simulink model "Simulink_multiterminal_HVDC_grid_alphas"  (R2016a)
settings: Solver=ode4  StartTime=0.0  StopTime=tsimul  FixedStep=1e-5  MaxStep=1e-4  RelTol=1e-5
values from neighbouring files (symbols this model uses):
  c = 0.1616*(10^-6)    (= 1.616e-07)    [Parameters_multiterminal_HVDC_alphas.m]
  Cconv = 1.5*(10^-4)    (= 0.00015)    [Parameters_multiterminal_HVDC_alphas.m]
  d1 = 230    [Parameters_multiterminal_HVDC_alphas.m]
  d2 = 75    [Parameters_multiterminal_HVDC_alphas.m]
  d3 = 217    [Parameters_multiterminal_HVDC_alphas.m]
  E2ref = 640000    [Parameters_multiterminal_HVDC_alphas.m]
  Kp = 0.0017    [Parameters_multiterminal_HVDC_alphas.m]
  Kpdc1 = Kpdc*alpha    (= 0)    [Parameters_multiterminal_HVDC_alphas.m]
  Kpdc2 = Kpdc*(1-alpha)    (= 4000)    [Parameters_multiterminal_HVDC_alphas.m]
  l1 = 0.2644*(10^-3)    (= 0.0002644)    [Parameters_multiterminal_HVDC_alphas.m]
  l2 = 7.2865*(10^-3)    (= 0.0072865)    [Parameters_multiterminal_HVDC_alphas.m]
  l3 = 3.6198*(10^-3)    (= 0.0036198)    [Parameters_multiterminal_HVDC_alphas.m]
  Ll = 0.1956    [Parameters_multiterminal_HVDC_alphas.m]
  Qref = 0    [Parameters_multiterminal_HVDC_alphas.m]
  r1 = 0.1265    [Parameters_multiterminal_HVDC_alphas.m]
  r2 = 0.1504    [Parameters_multiterminal_HVDC_alphas.m]
  r3 = 0.0178    [Parameters_multiterminal_HVDC_alphas.m]
  Rg = (1/g)    (= 9852216.74877)    [Parameters_multiterminal_HVDC_alphas.m]
  rl = 3.072    [Parameters_multiterminal_HVDC_alphas.m]
  tau = 0.001    [Parameters_multiterminal_HVDC_alphas.m]
  taupll = 0.0045    [Parameters_multiterminal_HVDC_alphas.m]
  Uab = 320000    [Parameters_multiterminal_HVDC_alphas.m]
libraries: powerlib x115, simulink x4
(part 2 of 2)

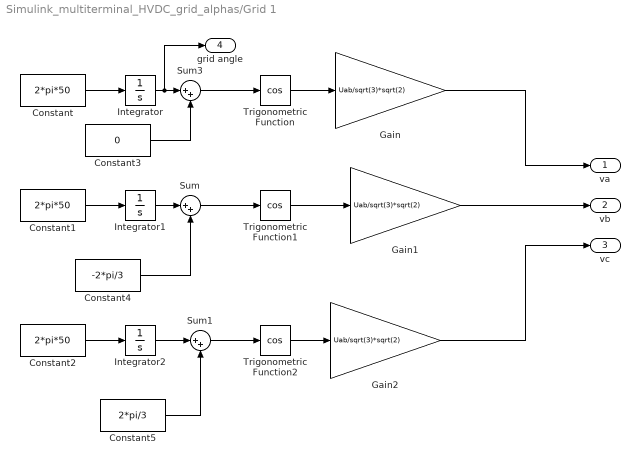
== system Simulink_multiterminal_HVDC_grid_alphas/Grid 1 ==
  Constant : Constant  Value=2*pi*50
  Constant1 : Constant  Value=2*pi*50
  Constant2 : Constant  Value=2*pi*50
  Constant3 : Constant  Value=0
  Constant4 : Constant  Value=-2*pi/3
  Constant5 : Constant  Value=2*pi/3
  Gain : Gain  Gain=Uab/sqrt(3)*sqrt(2)
  Gain1 : Gain  Gain=Uab/sqrt(3)*sqrt(2)
  Gain2 : Gain  Gain=Uab/sqrt(3)*sqrt(2)
  Integrator : Integrator
  Integrator1 : Integrator
  Integrator2 : Integrator
  Sum : Sum  Inputs=|++
  Sum1 : Sum  Inputs=|++
  Sum3 : Sum  Inputs=|++
  Trigonometric Function : Trigonometry  Operator=cos
  Trigonometric Function1 : Trigonometry  Operator=cos
  Trigonometric Function2 : Trigonometry  Operator=cos
  va : Outport
  vb : Outport  Port=2
  vc : Outport  Port=3
  grid angle : Outport  Port=4
  wires:
  Constant2/1 -> Integrator2/1
  Integrator2/1 -> Sum1/1
  Gain2/1 -> vc/1
  Sum1/1 -> Trigonometric Function2/1
  Sum3/1 -> Trigonometric Function/1
  Integrator/1 -> grid angle/1, Sum3/1
  Constant5/1 -> Sum1/2
  Constant4/1 -> Sum/2
  Integrator1/1 -> Sum/1
  Trigonometric Function/1 -> Gain/1
  Gain/1 -> va/1
  Constant1/1 -> Integrator1/1
  Trigonometric Function2/1 -> Gain2/1
  Constant/1 -> Integrator/1
  Constant3/1 -> Sum3/2
  Trigonometric Function1/1 -> Gain1/1
  Gain1/1 -> vb/1
  Sum/1 -> Trigonometric Function1/1

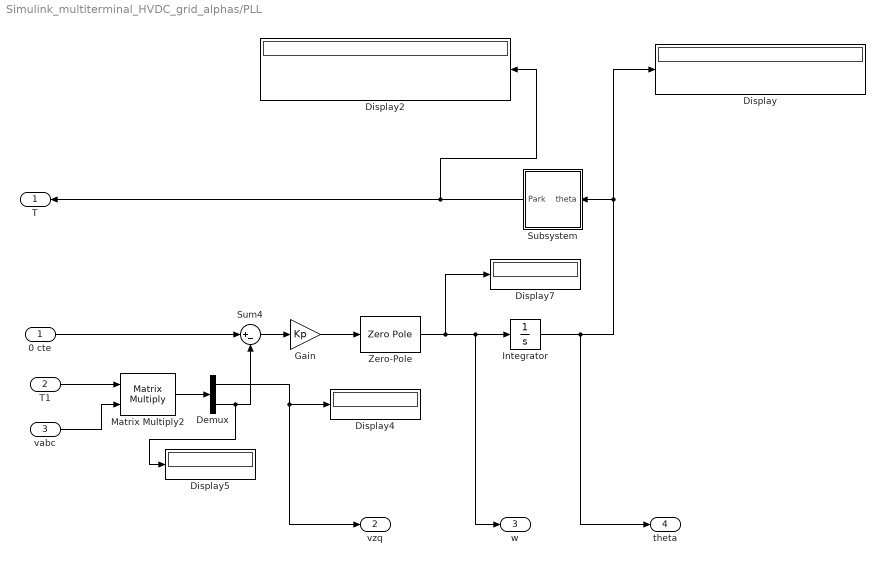
== system Simulink_multiterminal_HVDC_grid_alphas/PLL  ==
  0 cte : Inport
  T1 : Inport  Port=2
  vabc : Inport  Port=3
  Demux : Demux  Outputs=2
  Display{,2,4..5,7} (5 alike) : Display
  Gain : Gain  Gain=Kp
  Integrator : Integrator
  Matrix Multiply2 : Product  Multiplication=Matrix(*)
  Subsystem : Subsystem
  Sum4 : Sum  Inputs=|+-
  Zero-Pole : ZeroPole  Zeros=[-1/taupll]  Poles=[0]
  T : Outport
  vzq : Outport  Port=2
  w : Outport  Port=3
  theta : Outport  Port=4
  wires:
  0 cte/1 -> Sum4/1
  Subsystem/1(Park) -> T/1, Display2/1
  Sum4/1 -> Gain/1
  Gain/1 -> Zero-Pole/1
  Zero-Pole/1 -> Display7/1, w/1, Integrator/1
  Integrator/1 -> theta/1, Display/1, Subsystem/1(theta)
  T1/1 -> Matrix Multiply2/1
  vabc/1 -> Matrix Multiply2/2
  Matrix Multiply2/1 -> Demux/1
  Demux/2 -> Display5/1, Sum4/2
  Demux/1 -> vzq/1, Display4/1

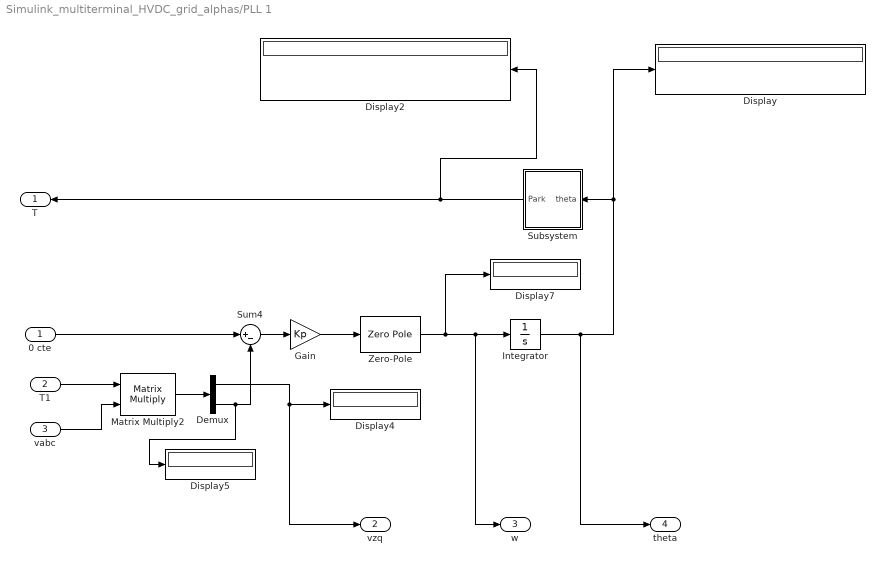
== system Simulink_multiterminal_HVDC_grid_alphas/PLL 1 ==
  0 cte : Inport
  T1 : Inport  Port=2
  vabc : Inport  Port=3
  Demux : Demux  Outputs=2
  Display{,2,4..5,7} (5 alike) : Display
  Gain : Gain  Gain=Kp
  Integrator : Integrator
  Matrix Multiply2 : Product  Multiplication=Matrix(*)
  Subsystem : Subsystem
  Sum4 : Sum  Inputs=|+-
  Zero-Pole : ZeroPole  Zeros=[-1/taupll]  Poles=[0]
  T : Outport
  vzq : Outport  Port=2
  w : Outport  Port=3
  theta : Outport  Port=4
  wires:
  0 cte/1 -> Sum4/1
  Subsystem/1(Park) -> T/1, Display2/1
  Sum4/1 -> Gain/1
  Gain/1 -> Zero-Pole/1
  Zero-Pole/1 -> Display7/1, w/1, Integrator/1
  Integrator/1 -> theta/1, Display/1, Subsystem/1(theta)
  T1/1 -> Matrix Multiply2/1
  vabc/1 -> Matrix Multiply2/2
  Matrix Multiply2/1 -> Demux/1
  Demux/2 -> Display5/1, Sum4/2
  Demux/1 -> vzq/1, Display4/1

== system Simulink_multiterminal_HVDC_grid_alphas/Pac ==
  iabc : Inport
  vabc : Inport  Port=2
  Add : Sum  Inputs=+++
  Demux3 : Demux  Outputs=3
  Demux4 : Demux  Outputs=3
  Display23 : Display
  Product7 : Product
  Product8 : Product
  Product9 : Product
  Pac : Outport
  wires:
  vabc/1 -> Demux4/1
  Product7/1 -> Add/1
  Demux3/1 -> Product7/1
  Demux3/3 -> Product8/1
  Product9/1 -> Add/2
  Add/1 -> Pac/1, Display23/1
  Demux4/3 -> Product8/2
  Demux3/2 -> Product9/1
  Product8/1 -> Add/3
  Demux4/1 -> Product7/2
  Demux4/2 -> Product9/2
  iabc/1 -> Demux3/1

== system Simulink_multiterminal_HVDC_grid_alphas/Pac1 ==
  iabc : Inport
  vabc : Inport  Port=2
  Add : Sum  Inputs=+++
  Demux3 : Demux  Outputs=3
  Demux4 : Demux  Outputs=3
  Display23 : Display
  Product7 : Product
  Product8 : Product
  Product9 : Product
  Pac : Outport
  wires:
  vabc/1 -> Demux4/1
  Product7/1 -> Add/1
  Demux3/1 -> Product7/1
  Demux3/3 -> Product8/1
  Product9/1 -> Add/2
  Add/1 -> Pac/1, Display23/1
  Demux4/3 -> Product8/2
  Demux3/2 -> Product9/1
  Product8/1 -> Add/3
  Demux4/1 -> Product7/2
  Demux4/2 -> Product9/2
  iabc/1 -> Demux3/1

== system Simulink_multiterminal_HVDC_grid_alphas/Pacc ==
  iabc : Inport
  vabcc : Inport  Port=2
  Add1 : Sum  Inputs=+++
  Demux5 : Demux  Outputs=3
  Demux6 : Demux  Outputs=3
  Display28 : Display
  Product10 : Product
  Product11 : Product
  Product12 : Product
  Pacc : Outport
  wires:
  iabc/1 -> Demux5/1
  Demux6/1 -> Product10/2
  Demux5/1 -> Product10/1
  vabcc/1 -> Demux6/1
  Demux6/2 -> Product12/2
  Demux5/2 -> Product12/1
  Demux6/3 -> Product11/2
  Demux5/3 -> Product11/1
  Product12/1 -> Add1/2
  Add1/1 -> Pacc/1, Display28/1
  Product11/1 -> Add1/3
  Product10/1 -> Add1/1

== system Simulink_multiterminal_HVDC_grid_alphas/Pacc1 ==
  iabc : Inport
  vabcc : Inport  Port=2
  Add1 : Sum  Inputs=+++
  Demux5 : Demux  Outputs=3
  Demux6 : Demux  Outputs=3
  Display28 : Display
  Product10 : Product
  Product11 : Product
  Product12 : Product
  Pacc : Outport
  wires:
  iabc/1 -> Demux5/1
  Demux6/1 -> Product10/2
  Demux5/1 -> Product10/1
  vabcc/1 -> Demux6/1
  Demux6/2 -> Product12/2
  Demux5/2 -> Product12/1
  Demux6/3 -> Product11/2
  Demux5/3 -> Product11/1
  Product12/1 -> Add1/2
  Add1/1 -> Pacc/1, Display28/1
  Product11/1 -> Add1/3
  Product10/1 -> Add1/1

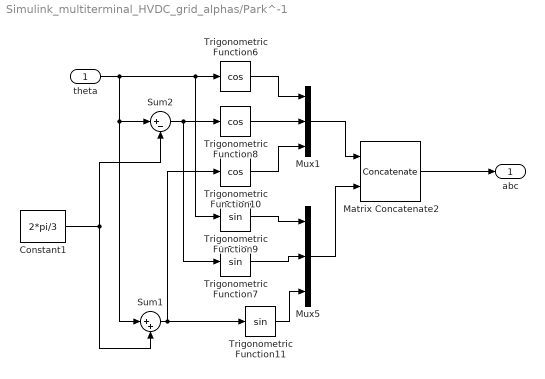
== system Simulink_multiterminal_HVDC_grid_alphas/Park^-1 ==
  theta : Inport  PortDimensions=1
  Constant1 : Constant  Value=2*pi/3  SampleTime=-1
  Matrix Concatenate2 : Concatenate  Mode=Multidimensional array  ConcatenateDimension=2
  Mux1 : Mux  Inputs=3
  Mux5 : Mux  Inputs=3
  Sum1 : Sum  Inputs=|++
  Sum2 : Sum  Inputs=|+-
  Trigonometric Function10 : Trigonometry  Operator=cos
  Trigonometric Function11 : Trigonometry
  Trigonometric Function6 : Trigonometry  Operator=cos
  Trigonometric Function7 : Trigonometry
  Trigonometric Function8 : Trigonometry  Operator=cos
  Trigonometric Function9 : Trigonometry
  abc : Outport
  wires:
  Trigonometric Function6/1 -> Mux1/1
  Sum1/1 -> Trigonometric Function10/1, Trigonometric Function11/1
  Sum2/1 -> Trigonometric Function7/1, Trigonometric Function8/1
  Mux1/1 -> Matrix Concatenate2/1
  Constant1/1 -> Sum2/2, Sum1/2
  theta/1 -> Trigonometric Function9/1, Trigonometric Function6/1, Sum2/1, Sum1/1
  Trigonometric Function11/1 -> Mux5/3
  Trigonometric Function9/1 -> Mux5/1
  Mux5/1 -> Matrix Concatenate2/2
  Trigonometric Function7/1 -> Mux5/2
  Matrix Concatenate2/1 -> abc/1
  Trigonometric Function8/1 -> Mux1/2
  Trigonometric Function10/1 -> Mux1/3

== system Simulink_multiterminal_HVDC_grid_alphas/Park^-2 ==
  theta : Inport  PortDimensions=1
  Constant1 : Constant  Value=2*pi/3  SampleTime=-1
  Matrix Concatenate2 : Concatenate  Mode=Multidimensional array  ConcatenateDimension=2
  Mux1 : Mux  Inputs=3
  Mux5 : Mux  Inputs=3
  Sum1 : Sum  Inputs=|++
  Sum2 : Sum  Inputs=|+-
  Trigonometric Function10 : Trigonometry  Operator=cos
  Trigonometric Function11 : Trigonometry
  Trigonometric Function6 : Trigonometry  Operator=cos
  Trigonometric Function7 : Trigonometry
  Trigonometric Function8 : Trigonometry  Operator=cos
  Trigonometric Function9 : Trigonometry
  abc : Outport
  wires:
  Trigonometric Function6/1 -> Mux1/1
  Sum1/1 -> Trigonometric Function10/1, Trigonometric Function11/1
  Sum2/1 -> Trigonometric Function7/1, Trigonometric Function8/1
  Mux1/1 -> Matrix Concatenate2/1
  Constant1/1 -> Sum2/2, Sum1/2
  theta/1 -> Trigonometric Function9/1, Trigonometric Function6/1, Sum2/1, Sum1/1
  Trigonometric Function11/1 -> Mux5/3
  Trigonometric Function9/1 -> Mux5/1
  Mux5/1 -> Matrix Concatenate2/2
  Trigonometric Function7/1 -> Mux5/2
  Matrix Concatenate2/1 -> abc/1
  Trigonometric Function8/1 -> Mux1/2
  Trigonometric Function10/1 -> Mux1/3

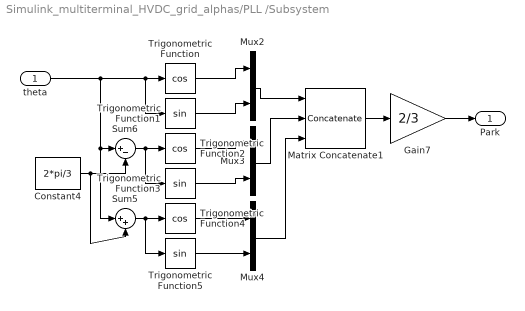
== system Simulink_multiterminal_HVDC_grid_alphas/PLL /Subsystem ==
  theta : Inport  PortDimensions=1
  Constant4 : Constant  Value=2*pi/3  SampleTime=-1
  Gain7 : Gain  Gain=2/3
  Matrix Concatenate1 : Concatenate  NumInputs=3  Mode=Multidimensional array  ConcatenateDimension=2
  Mux2 : Mux  Inputs=2
  Mux3 : Mux  Inputs=2
  Mux4 : Mux  Inputs=2
  Sum5 : Sum  Inputs=|++
  Sum6 : Sum  Inputs=|+-
  Trigonometric Function : Trigonometry  Operator=cos
  Trigonometric Function1 : Trigonometry
  Trigonometric Function2 : Trigonometry  Operator=cos
  Trigonometric Function3 : Trigonometry
  Trigonometric Function4 : Trigonometry  Operator=cos
  Trigonometric Function5 : Trigonometry
  Park : Outport
  wires:
  Trigonometric Function/1 -> Mux2/1
  Sum5/1 -> Trigonometric Function4/1, Trigonometric Function5/1
  Trigonometric Function3/1 -> Mux3/2
  Trigonometric Function2/1 -> Mux3/1
  Sum6/1 -> Trigonometric Function2/1, Trigonometric Function3/1
  Trigonometric Function1/1 -> Mux2/2
  Gain7/1 -> Park/1
  Matrix Concatenate1/1 -> Gain7/1
  Mux4/1 -> Matrix Concatenate1/3
  Mux3/1 -> Matrix Concatenate1/2
  Mux2/1 -> Matrix Concatenate1/1
  Trigonometric Function5/1 -> Mux4/2
  Trigonometric Function4/1 -> Mux4/1
  Constant4/1 -> Sum6/2, Sum5/2
  theta/1 -> Sum5/1, Sum6/1, Trigonometric Function/1, Trigonometric Function1/1

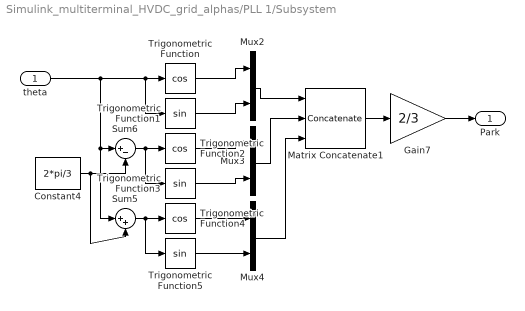
== system Simulink_multiterminal_HVDC_grid_alphas/PLL 1/Subsystem ==
  theta : Inport  PortDimensions=1
  Constant4 : Constant  Value=2*pi/3  SampleTime=-1
  Gain7 : Gain  Gain=2/3
  Matrix Concatenate1 : Concatenate  NumInputs=3  Mode=Multidimensional array  ConcatenateDimension=2
  Mux2 : Mux  Inputs=2
  Mux3 : Mux  Inputs=2
  Mux4 : Mux  Inputs=2
  Sum5 : Sum  Inputs=|++
  Sum6 : Sum  Inputs=|+-
  Trigonometric Function : Trigonometry  Operator=cos
  Trigonometric Function1 : Trigonometry
  Trigonometric Function2 : Trigonometry  Operator=cos
  Trigonometric Function3 : Trigonometry
  Trigonometric Function4 : Trigonometry  Operator=cos
  Trigonometric Function5 : Trigonometry
  Park : Outport
  wires:
  Trigonometric Function/1 -> Mux2/1
  Sum5/1 -> Trigonometric Function4/1, Trigonometric Function5/1
  Trigonometric Function3/1 -> Mux3/2
  Trigonometric Function2/1 -> Mux3/1
  Sum6/1 -> Trigonometric Function2/1, Trigonometric Function3/1
  Trigonometric Function1/1 -> Mux2/2
  Gain7/1 -> Park/1
  Matrix Concatenate1/1 -> Gain7/1
  Mux4/1 -> Matrix Concatenate1/3
  Mux3/1 -> Matrix Concatenate1/2
  Mux2/1 -> Matrix Concatenate1/1
  Trigonometric Function5/1 -> Mux4/2
  Trigonometric Function4/1 -> Mux4/1
  Constant4/1 -> Sum6/2, Sum5/2
  theta/1 -> Sum5/1, Sum6/1, Trigonometric Function/1, Trigonometric Function1/1
